simulink model "TST_EnumTypesStateflow"  (Simulink 10.0)
settings: Solver=FixedStepDiscrete  StartTime=0.0  StopTime=10.0  FixedStep=0.02  RelTol=1e-3  EnableMultiTasking=on
undefined symbols (not defined in the file): DIL_VmmGsFcsCommandsMessage_LatApModeCmd, DIL_VmmGsFcsCommandsMessage_LongApModeCmd
settings Model: Creator=kharthforeign  LastModifiedBy=unknown
settings DataIOCC: LimitDataPoints=on  SignalLoggingSaveFormat=ModelDataLogs  SaveOutput=off  SignalLogging=off  SaveTime=off
settings OptimizationCC: BlockReduction=off  ConditionallyExecuteInputs=off  OptimizeBlockIOStorage=off  BufferReuse=off  GlobalBufferReuse=off  ExpressionFolding=off  ExpressionDepthLimit=2147483647  LocalBlockOutputs=off  InitFltsAndDblsToZero=on  OptimizeDataStoreBuffers=off  BusAssignmentInplaceUpdate=off
settings DebuggingCC: SolverPrmCheckMsg=warning  FcnCallInpInsideContextMsg=warning  StateNameClashWarn=warning
settings SFSimCC: SimParseCustomCode=off
settings GRTTargetCC: GeneratePreprocessorConditionals=Disable all
settings ConfigComp: CovExternalEMLEnable=off

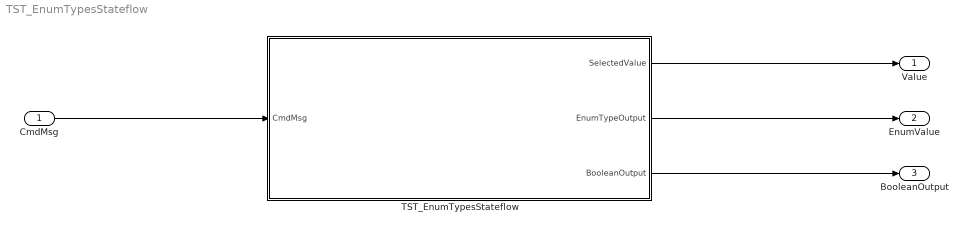
== system TST_EnumTypesStateflow ==
  CmdMsg : Inport  OutDataTypeStr=Bus: DIL_VmmGsFcsCommandsMessage_Data  BusOutputAsStruct=on
  TST_EnumTypesStateflow : Subsystem  TreatAsAtomicUnit=on
  Value : Outport  OutDataTypeStr=double  PortDimensions=1
  EnumValue : Outport  Port=2  OutDataTypeStr=Enum: DIL_VmmGsFcsCommandsMessage_LatApModeCmd  PortDimensions=1
  BooleanOutput : Outport  Port=3  OutDataTypeStr=boolean  PortDimensions=1
  wires:
  CmdMsg/1 -> TST_EnumTypesStateflow/1(CmdMsg)
  TST_EnumTypesStateflow/1(SelectedValue) -> Value/1
  TST_EnumTypesStateflow/2(EnumTypeOutput) -> EnumValue/1
  TST_EnumTypesStateflow/3(BooleanOutput) -> BooleanOutput/1

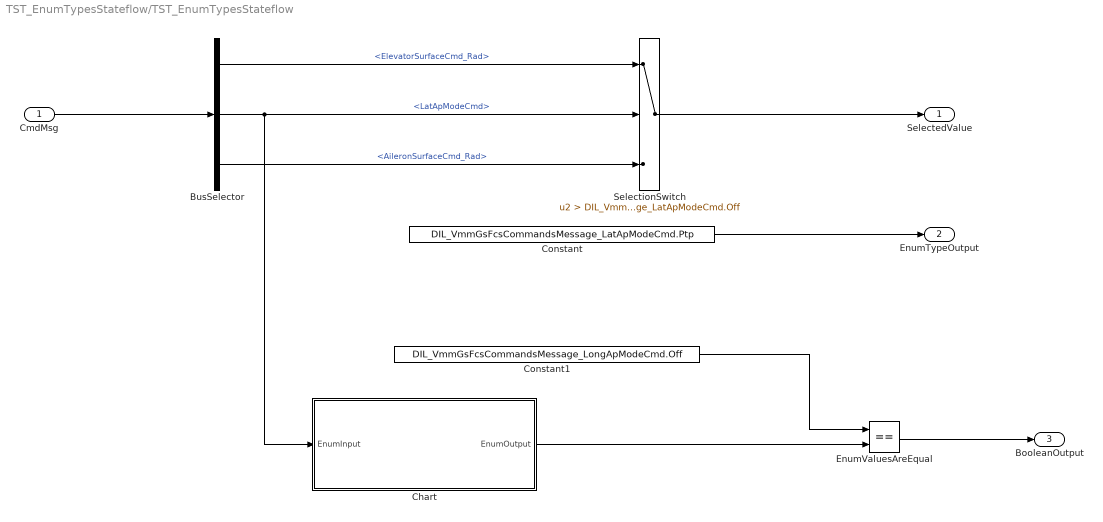
== system TST_EnumTypesStateflow/TST_EnumTypesStateflow ==
  CmdMsg : Inport  OutDataTypeStr=Bus: DIL_VmmGsFcsCommandsMessage_Data
  BusSelector : BusSelector  OutputSignals=ElevatorSurfaceCmd_Rad,LatApModeCmd,AileronSurfaceCmd_Rad
  Chart : Stateflow chart  TreatAsAtomicUnit=on
  Constant : Constant  Value=DIL_VmmGsFcsCommandsMessage_LatApModeCmd.Ptp  OutDataTypeStr=Enum: DIL_VmmGsFcsCommandsMessage_LatApModeCmd
  Constant1 : Constant  Value=DIL_VmmGsFcsCommandsMessage_LongApModeCmd.Off
  EnumValuesAreEqual : RelationalOperator  Operator===  OutDataTypeStr=boolean  RndMeth=Nearest
  SelectionSwitch : Switch  Criteria=u2 > Threshold  Threshold=DIL_VmmGsFcsCommandsMessage_LatApModeCmd.Off
  SelectedValue : Outport  OutDataTypeStr=double  PortDimensions=1
  EnumTypeOutput : Outport  Port=2  OutDataTypeStr=Enum: DIL_VmmGsFcsCommandsMessage_LatApModeCmd  PortDimensions=1
  BooleanOutput : Outport  Port=3  OutDataTypeStr=boolean  PortDimensions=1
  wires:
  CmdMsg/1 -> BusSelector/1
  SelectionSwitch/1 -> SelectedValue/1
  BusSelector/1 -> SelectionSwitch/1  "<ElevatorSurfaceCmd_Rad>"
  BusSelector/3 -> SelectionSwitch/3  "<AileronSurfaceCmd_Rad>"
  BusSelector/2 -> SelectionSwitch/2, Chart/1(EnumInput)  "<LatApModeCmd>"
  Constant/1 -> EnumTypeOutput/1
  Constant1/1 -> EnumValuesAreEqual/1
  Chart/1(EnumOutput) -> EnumValuesAreEqual/2
  EnumValuesAreEqual/1 -> BooleanOutput/1

== stateflow chart TST_EnumTypesStateflow/Chart ==
  state Ping
  state Pong
    entry:
    EnumOutput = ...
    DIL_VmmGsFcsCommandsMessage_LongApModeCmd.Altitude;
  (default) -> Ping
  Ping -> Pong : [EnumInput == ...
      |    DIL_VmmGsFcsCommandsMessage_LatApModeCmd.BankHeading]
  data: EnumInput input Enum: DIL_VmmGsFcsCommandsMessage_LatApModeCmd; EnumOutput output Enum: DIL_VmmGsFcsCommandsMessage_LongApModeCmd =DIL_VmmGsFcsCommandsMessage_LongApModeCmd.Off
